simulink model "Releroberto"  (R2021a)
settings: Solver=FixedStepAuto  StartTime=0.0  StopTime=1000  FixedStep=1e-4  RelTol=1e-3
settings Model: Creator=Royer  LastModifiedBy=Royer

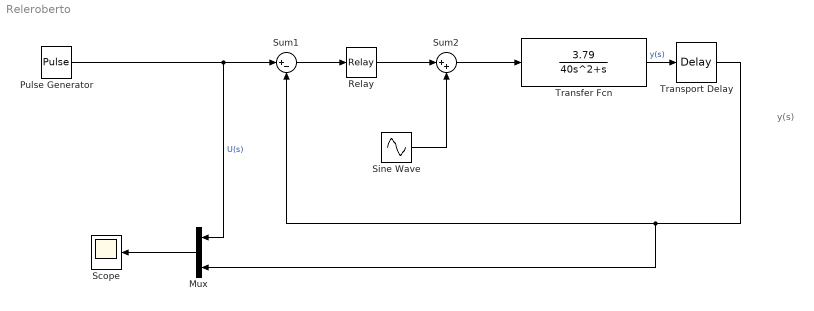
== system Releroberto ==
  note: y(s)
  Mux : Mux  Inputs=3
  Pulse Generator : DiscretePulseGenerator  PulseType=Time based  Amplitude=0.5  Period=50  PulseWidth=50
  Relay : Relay  OnSwitchValue=1  OffSwitchValue=-1  OffOutputValue=-1
  Scope : Scope
  Sine Wave : Sin  SampleTime=0
  Sum1 : Sum  Inputs=|+-
  Sum2 : Sum  Inputs=|++
  Transfer Fcn : TransferFcn  Numerator=[3.79]  Denominator=[40 1 0]
  Transport Delay : TransportDelay  DelayTime=2
  wires:
  Transfer Fcn/1 -> Transport Delay/1  "y(s)"
  Sum1/1 -> Relay/1
  Mux/1 -> Scope/1
  Pulse Generator/1 -> Mux/1, Sum1/1  "U(s)"
  Transport Delay/1 -> Mux/3, Sum1/2
  Relay/1 -> Sum2/1
  Sum2/1 -> Transfer Fcn/1
  Sine Wave/1 -> Sum2/2
